simulink model "Autotrans_shift_test"  (R2022a)
settings: Solver=VariableStepAuto  StartTime=0.0  StopTime=50.0  FixedStep=0.001  MinStep=0.0001  RelTol=1e-3
model workspace (MATLAB code in the model file):
  | load sldemo_autotrans_data; %load initial conditions and other necessary data
undefined symbols (not defined in the file or in its folder): converter_data, downtab, emap, Hecate_param1, Hecate_param2, Hecate_param3, Hecate_param4, Iei, uptab, vehicledata
settings Model: DataTypeOverride=Double  MinMaxOverflowLogging=ForceOff  SimulationMode=accelerator  ExtModeTrigMode=oneshot  ExtModeArmWhenConnect=off  LastModifiedBy=fedformi_new
settings DataIOCC: TimeSaveName=Time_output_test345
settings OptimizationCC: BlockReduction=off  BooleanDataType=off
settings DebuggingCC: SaveWithParameterizedLinksMsg=none  UnderspecifiedInitializationDetection=Classic  MergeDetectMultiDrivingBlocksExec=none  SignalResolutionControl=TryResolveAllWithWarning
settings HardwareCC: TargetUnknown=on
settings ModelReferenceCC: PropagateSignalLabelsOutOfModel=off

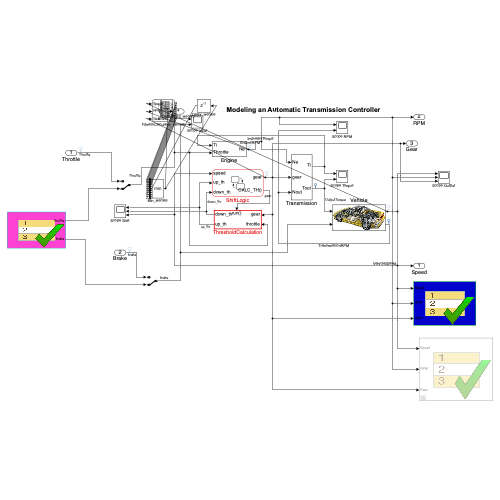
[thumbnail: Simulink's stored preview of the top-level diagram]
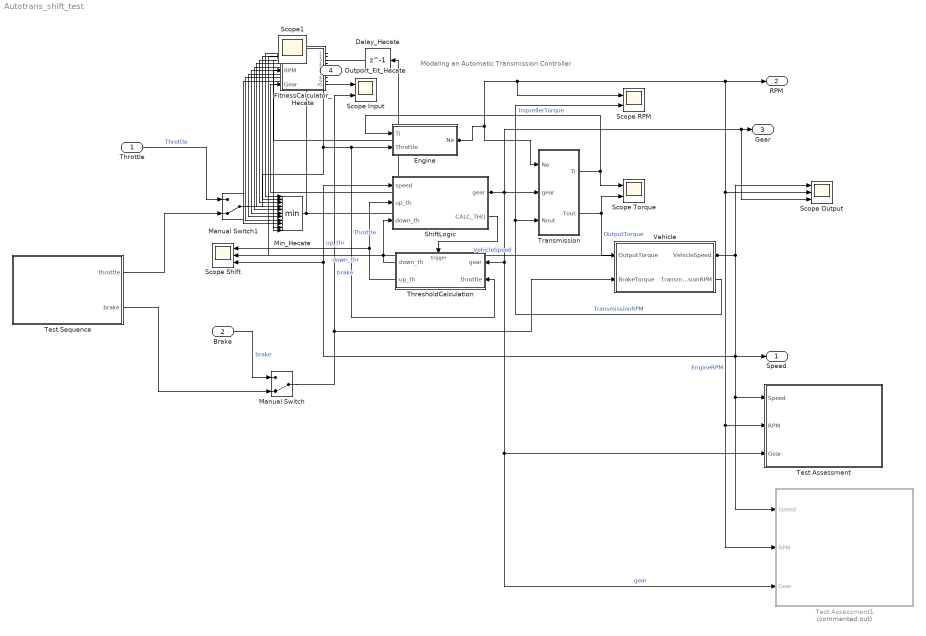
== system Autotrans_shift_test ==
  note: Modeling an Automatic Transmission Controller
  Throttle : Inport  Interpolate=off
  Brake : Inport  Port=2  Interpolate=off
  Delay_Hecate : Delay  DelayLength=1  InitialCondition=Inf
  Engine : Subsystem
  FitnessCalculator_Hecate : Stateflow chart  TreatAsAtomicUnit=on
  Manual Switch : ManualSwitch  CurrentSetting=0
  Manual Switch1 : ManualSwitch  CurrentSetting=0
  Min_Hecate : MinMax  Inputs=11
  Scope Input : Scope  NumInputPorts=2
  Scope Output : Scope  NumInputPorts=3
  Scope RPM : Scope  NumInputPorts=2
  Scope Shift : Scope  NumInputPorts=3
  Scope Torque : Scope  NumInputPorts=2
  ShiftLogic : Stateflow chart  TreatAsAtomicUnit=on
  Test Assessment : Test Sequence
  Test Assessment1 : Test Sequence  Commented=on  TreatAsAtomicUnit=on
  Test Sequence : Test Sequence  TreatAsAtomicUnit=on
  ThresholdCalculation : Subsystem  TreatAsAtomicUnit=on
  Transmission : Subsystem
  Vehicle : Subsystem  mask(vehicle model){Rfd=vehicledata(1), rload0=vehicledata(2), rload2=vehicledata(3), Rw=vehicledata(4), Iv=vehicledata(5), N20=vehicledata(6)/vehicledata(4)*vehicledata(1)}
      mask prompts: Rfd "final drive ratio"; rload0 "drag friction at wheels"; rload2 "aerodynamic drag"; Rw "wheel radius"; Iv "vehicle inertia"; N20 "initial transmission output speed"
      mask help: vehicle dynamics: torque input from trans., outputs are input speed (transmission output) and vehicle speed
      mask Display: image(imread([matlabroot,'/toolbox/simulink/simdemos/automotive/html/NSX_3Colors.jpg']))
  Speed : Outport  VectorParamsAs1DForOutWhenUnconnected=off
  RPM : Outport  Port=2  VectorParamsAs1DForOutWhenUnconnected=off
  Gear : Outport  Port=3  VectorParamsAs1DForOutWhenUnconnected=off
  Outport_Fit_Hecate : Outport  Port=4
  Scope1 : Scope
  wires:
  Transmission/1(Ti) -> Engine/1(Ti), Scope Torque/1  "ImprellerTorque"
  Engine/1(Ne) -> Transmission/1(Ne), Test Assessment1/2(RPM), Test Assessment/2(RPM), Scope Output/2, RPM/1, Scope RPM/1, FitnessCalculator_Hecate/2(RPM)  "EngineRPM"
  Vehicle/2(TransmissionRPM) -> Transmission/3(Nout), Scope RPM/2  "TransmissionRPM"
  ThresholdCalculation/1(down_th) -> Scope Shift/2, ShiftLogic/3(down_th)  "down_thr"
  ThresholdCalculation/2(up_th) -> ShiftLogic/2(up_th), Scope Shift/1  "up_thr"
  ShiftLogic/1(gear) -> ThresholdCalculation/1(gear), Test Assessment/3(Gear), Test Assessment1/3(Gear), Gear/1, Scope Output/3, Transmission/2(gear), FitnessCalculator_Hecate/3(Gear)  "gear"
  ShiftLogic/2(CALC_TH()) -> ThresholdCalculation/Trigger
  Vehicle/1(VehicleSpeed) -> Test Assessment1/1(Speed), Test Assessment/1(Speed), Speed/1, Scope Shift/3, ShiftLogic/1(speed), Scope Output/1, FitnessCalculator_Hecate/1(Speed)  "VehicleSpeed"
  Manual Switch1/1 -> ThresholdCalculation/2(throttle), Engine/2(Throttle), Scope Input/1  "Throttle"
  Transmission/2(Tout) -> Vehicle/1(OutputTorque), Scope Torque/2  "OutputTorque"
  Manual Switch/1 -> Vehicle/2(BrakeTorque), Scope Input/2  "brake"
  Test Sequence/1(throttle) -> Manual Switch1/2
  Test Sequence/2(brake) -> Manual Switch/2
  Brake/1 -> Manual Switch/1  "brake"
  Throttle/1 -> Manual Switch1/1  "Throttle"
  FitnessCalculator_Hecate/1(fitness_1) -> Min_Hecate/1
  FitnessCalculator_Hecate/2(fitness_2) -> Min_Hecate/2
  FitnessCalculator_Hecate/3(fitness_3) -> Min_Hecate/3
  FitnessCalculator_Hecate/4(fitness_4) -> Min_Hecate/4
  FitnessCalculator_Hecate/5(fitness_5) -> Min_Hecate/5
  FitnessCalculator_Hecate/6(fitness_6) -> Min_Hecate/6
  FitnessCalculator_Hecate/7(fitness_7) -> Min_Hecate/7
  FitnessCalculator_Hecate/8(fitness_8) -> Min_Hecate/8
  FitnessCalculator_Hecate/9(fitness_9) -> Min_Hecate/9
  FitnessCalculator_Hecate/10(fitness_10) -> Min_Hecate/10
  Min_Hecate/1 -> Delay_Hecate/1, Outport_Fit_Hecate/1
  Delay_Hecate/1 -> Min_Hecate/11

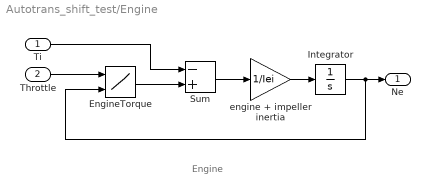
== system Autotrans_shift_test/Engine ==
  note: Engine
  Ti : Inport
  Throttle : Inport  Port=2
  EngineTorque : Lookup2D  RowIndex=thvec  ColumnIndex=nevec  Table=emap  SaturateOnIntegerOverflow=off
  Integrator : Integrator  InitialCondition=1000  LimitOutput=on  UpperSaturationLimit=6000  LowerSaturationLimit=600  ZeroCross=off
  Sum : Sum  Inputs=-+  InputSameDT=on  SaturateOnIntegerOverflow=on  OutDataTypeStr=Inherit: Same as first input
  engine + impeller inertia : Gain  Gain=1/Iei  SaturateOnIntegerOverflow=on  OutDataTypeStr=Inherit: Same as input  ParamDataTypeStr=Inherit: Same as input
  Ne : Outport  InitialOutput=0  VectorParamsAs1DForOutWhenUnconnected=off
  wires:
  Ti/1 -> Sum/1
  Throttle/1 -> EngineTorque/1
  Integrator/1 -> EngineTorque/2, Ne/1
  Sum/1 -> engine + impeller inertia/1
  engine + impeller inertia/1 -> Integrator/1
  EngineTorque/1 -> Sum/2

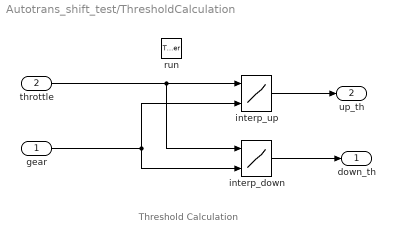
== system Autotrans_shift_test/ThresholdCalculation ==
  note: Threshold Calculation
  gear : Inport
  throttle : Inport  Port=2
  run : TriggerPort  TriggerType=function-call  VariantControl=(inherit)  ZeroCross=off
  interp_down : Lookup2D  RowIndex=downth  ColumnIndex=[1:4]  Table=downtab  OutDataTypeStr=double  SaturateOnIntegerOverflow=off  InputSameDT=off
      settings: LockScale=on
  interp_up : Lookup2D  RowIndex=upth  ColumnIndex=[1:4]  Table=uptab  OutDataTypeStr=double  SaturateOnIntegerOverflow=off  InputSameDT=off
      settings: LockScale=on
  down_th : Outport  VectorParamsAs1DForOutWhenUnconnected=off
  up_th : Outport  Port=2  VectorParamsAs1DForOutWhenUnconnected=off
  wires:
  interp_up/1 -> up_th/1
  interp_down/1 -> down_th/1
  throttle/1 -> interp_up/1, interp_down/1
  gear/1 -> interp_up/2, interp_down/2

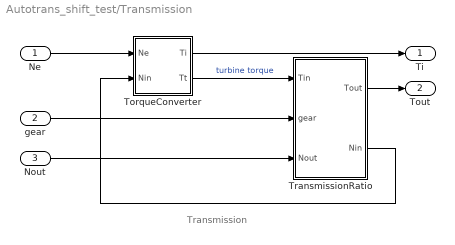
== system Autotrans_shift_test/Transmission ==
  note: Transmission
  Ne : Inport
  gear : Inport  Port=2
  Nout : Inport  Port=3
  TorqueConverter : Subsystem  mask(torque converter){speedratio=converter_data(:,1), Kfactor=converter_data(:,2), Torkratio=converter_data(:,3)}
      mask prompts: speedratio "speed ratio"; Kfactor "K factor"; Torkratio "torque ratio"
      mask help: torque converter
      mask Help: Torque converter input and output torques are computed as a function of the input and output speeds
      mask Display: plot([cos([90:10:450]*pi/180),.63*cos([90:10:450]*pi/180),.63*cos([90:10:240]*pi/180),cos([240:10:300]*pi/180),.63*cos([300]*pi/180)],[sin([90:10:450]*pi/180),.63*sin([90:10:450]*pi/180)+.1,.63*sin([90:10:240]*pi/180)+.1,sin([240:10:300]*pi/180),.63*sin([300]*pi/180)+.1])
  TransmissionRatio : Subsystem
  Ti : Outport  InitialOutput=0  VectorParamsAs1DForOutWhenUnconnected=off
  Tout : Outport  Port=2  InitialOutput=0  VectorParamsAs1DForOutWhenUnconnected=off
  wires:
  TransmissionRatio/1(Tout) -> Tout/1
  TorqueConverter/1(Ti) -> Ti/1
  Nout/1 -> TransmissionRatio/3(Nout)
  gear/1 -> TransmissionRatio/2(gear)
  Ne/1 -> TorqueConverter/1(Ne)
  TransmissionRatio/2(Nin) -> TorqueConverter/2(Nin)
  TorqueConverter/2(Tt) -> TransmissionRatio/1(Tin)  "turbine torque"

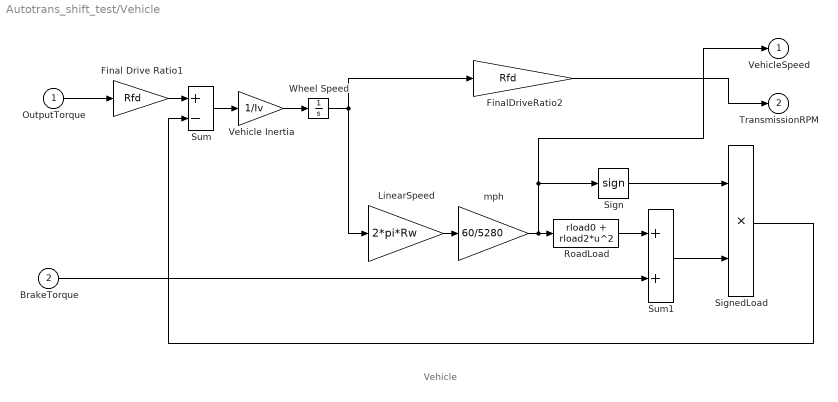
== system Autotrans_shift_test/Vehicle ==
  note: Vehicle
  OutputTorque : Inport
  BrakeTorque : Inport  Port=2
  Final Drive Ratio1 : Gain  Gain=Rfd  SaturateOnIntegerOverflow=on  OutDataTypeStr=Inherit: Same as input  ParamDataTypeStr=Inherit: Same as input
  FinalDriveRatio2 : Gain  Gain=Rfd  SaturateOnIntegerOverflow=on  OutDataTypeStr=Inherit: Same as input  ParamDataTypeStr=Inherit: Same as input
  LinearSpeed : Gain  Gain=2*pi*Rw  SaturateOnIntegerOverflow=on  OutDataTypeStr=Inherit: Same as input  ParamDataTypeStr=Inherit: Same as input
  RoadLoad : Fcn  Expr=rload0 + rload2*u^2
  Sign : Signum
  SignedLoad : Product  InputSameDT=on  SaturateOnIntegerOverflow=on  OutDataTypeStr=Inherit: Same as first input
  Sum : Sum  Inputs=+-  InputSameDT=on  SaturateOnIntegerOverflow=on  OutDataTypeStr=Inherit: Same as first input
  Sum1 : Sum  InputSameDT=on  SaturateOnIntegerOverflow=on  OutDataTypeStr=Inherit: Same as first input
  Vehicle Inertia : Gain  Gain=1/Iv  SaturateOnIntegerOverflow=on  OutDataTypeStr=Inherit: Same as input  ParamDataTypeStr=Inherit: Same as input
  Wheel Speed : Integrator  InitialCondition=N20/Rfd  ZeroCross=off
  mph : Gain  Gain=60/5280  SaturateOnIntegerOverflow=on  OutDataTypeStr=Inherit: Same as input  ParamDataTypeStr=Inherit: Same as input
  VehicleSpeed : Outport  InitialOutput=0  VectorParamsAs1DForOutWhenUnconnected=off
  TransmissionRPM : Outport  Port=2  InitialOutput=0  VectorParamsAs1DForOutWhenUnconnected=off
  wires:
  FinalDriveRatio2/1 -> TransmissionRPM/1
  BrakeTorque/1 -> Sum1/2
  Sum1/1 -> SignedLoad/2
  RoadLoad/1 -> Sum1/1
  Sign/1 -> SignedLoad/1
  SignedLoad/1 -> Sum/2
  OutputTorque/1 -> Final Drive Ratio1/1
  Vehicle Inertia/1 -> Wheel Speed/1
  Sum/1 -> Vehicle Inertia/1
  mph/1 -> VehicleSpeed/1, Sign/1, RoadLoad/1
  LinearSpeed/1 -> mph/1
  Wheel Speed/1 -> LinearSpeed/1, FinalDriveRatio2/1
  Final Drive Ratio1/1 -> Sum/1

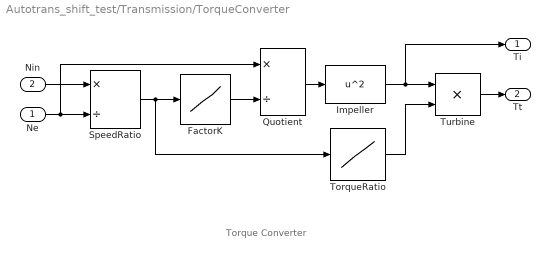
== system Autotrans_shift_test/Transmission/TorqueConverter ==
  note: Torque Converter
  Ne : Inport
  Nin : Inport  Port=2
  FactorK : Lookup  InputValues=speedratio  Table=Kfactor
  Impeller : Fcn  Expr=u^2
  Quotient : Product  Inputs=*/  InputSameDT=on  SaturateOnIntegerOverflow=on  OutDataTypeStr=Inherit: Same as first input
  SpeedRatio : Product  Inputs=*/  InputSameDT=on  SaturateOnIntegerOverflow=on  OutDataTypeStr=Inherit: Same as first input
  TorqueRatio : Lookup  InputValues=speedratio  Table=Torkratio
  Turbine : Product  InputSameDT=on  SaturateOnIntegerOverflow=on  OutDataTypeStr=Inherit: Same as first input
  Ti : Outport  InitialOutput=0  VectorParamsAs1DForOutWhenUnconnected=off
  Tt : Outport  Port=2  InitialOutput=0  VectorParamsAs1DForOutWhenUnconnected=off
  wires:
  TorqueRatio/1 -> Turbine/2
  Quotient/1 -> Impeller/1
  FactorK/1 -> Quotient/2
  SpeedRatio/1 -> TorqueRatio/1, FactorK/1
  Impeller/1 -> Turbine/1, Ti/1
  Turbine/1 -> Tt/1
  Ne/1 -> SpeedRatio/2, Quotient/1
  Nin/1 -> SpeedRatio/1

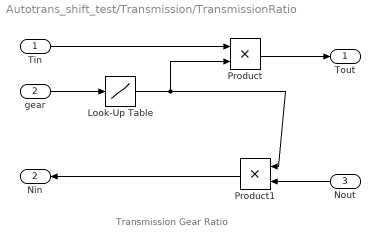
== system Autotrans_shift_test/Transmission/TransmissionRatio ==
  note: Transmission Gear Ratio
  Tin : Inport
  gear : Inport  Port=2
  Nout : Inport  Port=3
  Look-Up Table : Lookup  InputValues=[1 2 3 4]  Table=[2.393 1.450 1.000 0.677]  OutDataTypeStr=double  LockScale=on
  Product : Product  InputSameDT=on  SaturateOnIntegerOverflow=on  OutDataTypeStr=Inherit: Same as first input
  Product1 : Product  InputSameDT=on  SaturateOnIntegerOverflow=on  OutDataTypeStr=Inherit: Same as first input
  Tout : Outport  InitialOutput=0  VectorParamsAs1DForOutWhenUnconnected=off
  Nin : Outport  Port=2  InitialOutput=0  VectorParamsAs1DForOutWhenUnconnected=off
  wires:
  Look-Up Table/1 -> Product1/1, Product/2
  Nout/1 -> Product1/2
  Product1/1 -> Nin/1
  Product/1 -> Tout/1
  Tin/1 -> Product/1
  gear/1 -> Look-Up Table/1

== stateflow chart Autotrans_shift_test/Test Assessment1 ==
  state step_1
    verify(Speed >= 20)
    state step_1_1
      verify(Speed <= 30)
    state step_1_2
      verify(Speed <= 60)
    state step_1_3
      verify(1<=1)
      state step_1_3_1
        verify(Speed <= 80)
      state step_1_3_2
        verify(Speed <= 90)
        verify(Speed*30 >= RPM)
      state step_1_3_3
        verify(Speed <= 100)
        state step_1_3_2_1
          verify(Speed/20 > RPM/1000-Gear)
        state step_1_3_2_2
          verify(Speed/20 < RPM/1000+Gear)
        (default) -> (junction 99)
        step_1_3_3 -> (junction 99)
        (junction 99) -> (junction 100) [order 1] : [Speed <= 60
            | ]
        (junction 100) -> step_1_3_2_1 [order 1] : [~in(step_1.step_1_3.step_1_3_3.step_1_3_2_1)]
        (junction 100) -> (junction 103) [order 2]
        (junction 109) -> (junction 110)
        (junction 110) -> step_1_3_2_2 [order 1] : [~in(step_1.step_1_3.step_1_3_3.step_1_3_2_2)]
        (junction 110) -> (junction 113) [order 2]
        (junction 99) -> (junction 109) [order 2]
      (junction 91) -> (junction 94) [order 2]
      (junction 82) -> (junction 90) [order 2]
      (default) -> (junction 73)
      step_1_3 -> (junction 73)
      (junction 73) -> (junction 74) [order 1] : [RPM <= 3000
          | ]
      (junction 74) -> step_1_3_1 [order 1] : [~in(step_1.step_1_3.step_1_3_1)]
      (junction 73) -> (junction 82) [order 2]
      (junction 74) -> (junction 77) [order 2]
      (junction 82) -> (junction 83) [order 1] : [RPM <= 4000
          | ]
      (junction 83) -> step_1_3_2 [order 1] : [~in(step_1.step_1_3.step_1_3_2)]
      (junction 83) -> (junction 86) [order 2]
      (junction 90) -> (junction 91)
      (junction 91) -> step_1_3_3 [order 1] : [~in(step_1.step_1_3.step_1_3_3)]
    state step_1_4
      verify(Speed <= 150)
    step_1 -> (junction 47)
    (default) -> (junction 47)
    (junction 47) -> (junction 48) [order 1] : [Gear == 1
        | ]
    (junction 48) -> step_1_1 [order 1] : [~in(step_1.step_1_1)]
    (junction 47) -> (junction 56) [order 2]
    (junction 48) -> (junction 51) [order 2]
    (junction 56) -> (junction 57) [order 1] : [Gear == 2
        | ]
    (junction 57) -> step_1_2 [order 1] : [~in(step_1.step_1_2)]
    (junction 56) -> (junction 64) [order 2]
    (junction 57) -> (junction 60) [order 2]
    (junction 64) -> (junction 65) [order 1] : [Gear == 3
        | ]
    (junction 65) -> step_1_3 [order 1] : [~in(step_1.step_1_3)]
    (junction 65) -> (junction 68) [order 2]
    (junction 117) -> (junction 118)
    (junction 118) -> step_1_4 [order 1] : [~in(step_1.step_1_4)]
    (junction 118) -> (junction 121) [order 2]
    (junction 64) -> (junction 117) [order 2]
  (default) -> step_1
  data: Speed input; RPM input; Gear input

== stateflow chart Autotrans_shift_test/Test Sequence ==
  state Accelerate
    throttle = 100-Hecate_param1;
    % Random comment;
    brake = 0+Hecate_param2;
  state Constant_speed
    throttle = 0;
    brake = 0+Hecate_param4;
  (default) -> Accelerate
  Accelerate -> Constant_speed : [
      | after(20-Hecate_param3,sec)
      | ]
  data: throttle output; brake output; Hecate_param1 parameter; Hecate_param2 parameter; Hecate_param3 parameter; Hecate_param4 parameter

== stateflow chart Autotrans_shift_test/FitnessCalculator_Hecate ==
  state step_1
    fitness_1 = Inf;
    fitness_2 = Inf;
    fitness_3 = Inf;
    fitness_4 = Inf;
    fitness_5 = Inf;
    fitness_6 = Inf;
    fitness_7 = Inf;
    fitness_8 = Inf;
    fitness_9 = Inf;
    fitness_10 = Inf;
    state step_1_1
      fitness_1 = min([3000-(RPM);2-(Gear);Speed-(70);]);
      fitness_2 = max([70-(Speed);Gear-(3);Speed-(45);]);
      fitness_3 = Inf;
      fitness_4 = Inf;
      fitness_5 = Inf;
      fitness_6 = Inf;
      fitness_7 = Inf;
      fitness_8 = Inf;
      fitness_9 = Inf;
      fitness_10 = Inf;
      state step_1_1_1
        fitness_1 = min([3000-(RPM);2-(Gear);Speed-(70);]);
        fitness_2 = max([70-(Speed);Gear-(3);Speed-(45);]);
        fitness_3 = 50-(Speed);
        fitness_4 = Inf;
        fitness_5 = Inf;
        fitness_6 = Inf;
        fitness_7 = Inf;
        fitness_8 = Inf;
        fitness_9 = Inf;
        fitness_10 = Inf;
      state step_1_1_2
        fitness_1 = min([3000-(RPM);2-(Gear);Speed-(70);]);
        fitness_2 = max([70-(Speed);Gear-(3);Speed-(45);]);
        fitness_3 = Inf;
        fitness_4 = Speed-(60);
        fitness_5 = Inf;
        fitness_6 = Inf;
        fitness_7 = Inf;
        fitness_8 = Inf;
        fitness_9 = Inf;
        fitness_10 = Inf;
      (default) -> step_1_1_1
      step_1_1_2 -> step_1_1_1 : [RPM < 2900]
      step_1_1_1 -> step_1_1_2 : [RPM >= 3300]
    state step_1_2
      fitness_1 = Inf;
      fitness_2 = Inf;
      fitness_3 = Inf;
      fitness_4 = Inf;
      fitness_5 = 3500-(RPM);
      fitness_6 = Inf;
      fitness_7 = Inf;
      fitness_8 = Inf;
      fitness_9 = Inf;
      fitness_10 = Inf;
    state step_1_3
      fitness_1 = Inf;
      fitness_2 = Inf;
      fitness_3 = Inf;
      fitness_4 = Inf;
      fitness_5 = Inf;
      fitness_6 = 4000-(RPM);
      fitness_7 = Inf;
      fitness_8 = Inf;
      fitness_9 = Inf;
      fitness_10 = Inf;
    (default) -> (junction 4)
    step_1_3 -> (junction 4) : [(Gear <= 2)|(Gear == 3)]
    step_1_2 -> (junction 4) : [(Gear <= 2)|~(Gear == 3)]
    (junction 4) -> step_1_1 [order 1] : [Gear <= 2]
    (junction 4) -> step_1_2 [order 2] : [Gear == 3]
    (junction 4) -> step_1_3 [order 3] : []
    step_1_1 -> (junction 4) : [~(Gear <= 2)]
  state step_2
    fitness_1 = Inf;
    fitness_2 = Inf;
    fitness_3 = Inf;
    fitness_4 = Inf;
    fitness_5 = Inf;
    fitness_6 = Inf;
    fitness_7 = Inf;
    fitness_8 = Inf;
    fitness_9 = Inf;
    fitness_10 = Inf;
    state step_2_2
      fitness_1 = Inf;
      fitness_2 = Inf;
      fitness_3 = Inf;
      fitness_4 = Inf;
      fitness_5 = Inf;
      fitness_6 = Inf;
      fitness_7 = Inf;
      fitness_8 = Inf;
      fitness_9 = Inf;
      fitness_10 = Inf;
      state step_2_2_1
        fitness_1 = Inf;
        fitness_2 = Inf;
        fitness_3 = Inf;
        fitness_4 = Inf;
        fitness_5 = Inf;
        fitness_6 = Inf;
        fitness_7 = Inf;
        fitness_8 = 100-(Speed);
        fitness_9 = Inf;
        fitness_10 = Inf;
      state step_2_2_2
        fitness_1 = Inf;
        fitness_2 = Inf;
        fitness_3 = Inf;
        fitness_4 = Inf;
        fitness_5 = Inf;
        fitness_6 = Inf;
        fitness_7 = Inf;
        fitness_8 = Inf;
        fitness_9 = Speed-(110);
        fitness_10 = Inf;
      (default) -> (junction 22)
      step_2_2_2 -> (junction 22) : [(RPM < 3700)]
      step_2_2_1 -> (junction 22) : [~(RPM < 3700)]
      (junction 22) -> step_2_2_1 [order 1] : [RPM < 3700]
      (junction 22) -> step_2_2_2 [order 2] : []
    state step_2_1
      fitness_1 = Inf;
      fitness_2 = Inf;
      fitness_3 = Inf;
      fitness_4 = Inf;
      fitness_5 = Inf;
      fitness_6 = Inf;
      fitness_7 = 90-(Speed);
      fitness_8 = Inf;
      fitness_9 = Inf;
      fitness_10 = Inf;
    (default) -> step_2_1
    step_2_2 -> step_2_1 : [true]
    step_2_1 -> step_2_2 : [after(2, sec) && Gear == 4]
  state step_3
    fitness_1 = Inf;
    fitness_2 = Inf;
    fitness_3 = Inf;
    fitness_4 = Inf;
    fitness_5 = Inf;
    fitness_6 = Inf;
    fitness_7 = Inf;
    fitness_8 = Inf;
    fitness_9 = Inf;
    fitness_10 = Speed-(70);
  (default) -> step_1
  step_1 -> step_3 [order 1] : [Speed > 120]
  step_1 -> step_2 [order 2] : [after(25, sec)]
  step_2 -> step_3 : [after(20, sec)]
  data: Speed input; RPM input; Gear input; fitness_1 output; fitness_2 output; fitness_3 output; fitness_4 output; fitness_5 output; fitness_6 output; fitness_7 output; fitness_8 output; fitness_9 output; fitness_10 output

== stateflow chart Autotrans_shift_test/ShiftLogic ==
  settings: updateMethod=DISCRETE  sampleTime=0.04
  state gear_state [parallel]
    settings: executionOrder=1
    state fourth
      entry:
      gear = 4;
    state third
      entry:
      gear = 3;
    state second
      entry:
      gear = 2;
    state first
      entry:
      gear = 1;
    (default) -> first
    second -> third [order 1] : UP
    first -> second : UP
    third -> fourth [order 1] : UP
    second -> first [order 2] : DOWN
    fourth -> third : DOWN
    third -> second [order 2] : DOWN
  state selection_state [parallel]
    during: CALC_TH;
    settings: executionOrder=2
    state steady_state
    state upshifting
    state downshifting
    (default) -> steady_state
    steady_state -> upshifting [order 1] : [speed > up_th]
    steady_state -> downshifting [order 2] : [speed < down_th]
    downshifting -> steady_state [order 1] : after(TWAIT,tick)
        | [speed <= down_th]
        | {gear_state.DOWN}
    downshifting -> steady_state [order 2] : [speed > down_th]
    upshifting -> steady_state [order 1] : after(TWAIT,tick)
        | [speed >= up_th]
        | {gear_state.UP}
    upshifting -> steady_state [order 2] : [speed < up_th]
  data: speed input double; gear output fixdt(0,8,5) [1..4]; TWAIT parameter fixdt(0,8,6); up_th input double; down_th input double
  events: DOWN local EITHER_EDGE_EVENT; UP local EITHER_EDGE_EVENT; CALC_TH output FUNCTION_CALL_EVENT

== stateflow chart Autotrans_shift_test/Test Assessment ==
  state Scenario_1
    state Group1
      verify(Speed >= 0)
      state AT2
        verify(Speed < 120)
        state AT2_1
          verify(RPM<6000)
          verify(Speed >= 35)
        (default) -> AT2_1
      state ATend
        verify(Gear < 5)
      (junction 118) -> (junction 121) [order 2]
      (junction 108) -> (junction 117) [order 2]
      (default) -> (junction 108)
      Group1 -> (junction 108) [order 1]
      (junction 108) -> (junction 109) [order 1] : [RPM > 2500
          | ]
      (junction 109) -> AT2 [order 1] : [~in(Scenario_1.Group1.AT2)]
      (junction 109) -> (junction 112) [order 2]
      (junction 117) -> (junction 118)
      (junction 118) -> ATend [order 1] : [~in(Scenario_1.Group1.ATend)]
    state Group2
      verify(RPM >= 600)
    state Group3
      verify(Gear >= 0)
    (default) -> Group1
    Group1 -> (junction 564) [order 2] : [
        | t >= 10 && Gear >= 4
        | ]
    (junction 564) -> (junction 170)
    Group1 -> Group2 [order 1] : [
        | t >= 20
        | ]
    (junction 170) -> Group3
  state Scenario_2
    state step_1
      state step_1_1
        state step_1_1_1
          verify(RPM > 3000)
        state step_1_1_2
        (default) -> (junction 587)
        Scenario_2.step_1.step_1_1 -> (junction 587)
        (junction 587) -> (junction 588) [order 1] : [Speed-(RPM/1000)^Gear > 35 || t < 20
            | ]
        (junction 588) -> Scenario_2.step_1.step_1_1.step_1_1_1 [order 1] : [~in(Scenario_2.step_1.step_1_1.step_1_1_1)]
        (junction 588) -> (junction 591) [order 2]
        (junction 596) -> (junction 597)
        (junction 597) -> Scenario_2.step_1.step_1_1.step_1_1_2 [order 1] : [~in(Scenario_2.step_1.step_1_1.step_1_1_2)]
        (junction 597) -> (junction 600) [order 2]
        (junction 587) -> (junction 596) [order 2]
      state step_1_2
      (default) -> (junction 573)
      Scenario_2.step_1 -> (junction 573)
      (junction 573) -> (junction 574) [order 1] : [Speed <= 70 && hasChangedTo(Gear,2)
          | ]
      (junction 574) -> Scenario_2.step_1.step_1_1 [order 1] : [~in(Scenario_2.step_1.step_1_1)]
      (junction 574) -> (junction 577) [order 2]
      (junction 604) -> (junction 605)
      (junction 605) -> Scenario_2.step_1.step_1_2 [order 1] : [~in(Scenario_2.step_1.step_1_2)]
      (junction 605) -> (junction 608) [order 2]
      (junction 573) -> (junction 604) [order 2]
    (default) -> Scenario_2.step_1
  state Scenario_3
    state step_1
      state step_1_1
        verify(RPM < 3000 && Gear <= 2 & Speed > 70) % Random comment
        verify(Speed < 70 || Gear > 3 || Speed > 45)
        state step_1_1_1
          verify(Speed < 50)
        state step_1_1_2
          verify(Speed >= 60)
        (default) -> Scenario_3.step_1.step_1_1.step_1_1_1
        Scenario_3.step_1.step_1_1.step_1_1_1 -> Scenario_3.step_1.step_1_1.step_1_1_2 : [
            | RPM >= 3300
            | ]
        Scenario_3.step_1.step_1_1.step_1_1_2 -> Scenario_3.step_1.step_1_1.step_1_1_1 : [
            | RPM < 2900
            | ]
      state step_1_2
        verify(RPM <= 3500)
      state step_1_3
        verify(RPM < 4000)
      (default) -> (junction 206)
      Scenario_3.step_1 -> (junction 206) [order 1]
      (junction 206) -> (junction 207) [order 1] : [Gear <= 2
          | ]
      (junction 207) -> Scenario_3.step_1.step_1_1 [order 1] : [~in(Scenario_3.step_1.step_1_1)]
      (junction 206) -> (junction 223) [order 2]
      (junction 207) -> (junction 210) [order 2]
      (junction 223) -> (junction 224) [order 1] : [Gear == 3
          | ]
      (junction 224) -> Scenario_3.step_1.step_1_2 [order 1] : [~in(Scenario_3.step_1.step_1_2)]
      (junction 223) -> (junction 231) [order 2]
      (junction 224) -> (junction 227) [order 2]
      (junction 231) -> (junction 232)
      (junction 232) -> Scenario_3.step_1.step_1_3 [order 1] : [~in(Scenario_3.step_1.step_1_3)]
      (junction 232) -> (junction 235) [order 2]
    state step_2
      state step_2_1
        verify(Speed < 90)
      state step_2_2
        state step_2_2_1
          verify(Speed < 100)
        state step_2_2_2
          verify(Speed >= 110)
        (default) -> (junction 248)
        Scenario_3.step_2.step_2_2 -> (junction 248) [order 1]
        (junction 248) -> (junction 249) [order 1] : [RPM < 3700
            | ]
        (junction 249) -> Scenario_3.step_2.step_2_2.step_2_2_1 [order 1] : [~in(Scenario_3.step_2.step_2_2.step_2_2_1)]
        (junction 249) -> (junction 252) [order 2]
        (junction 257) -> (junction 258)
        (junction 258) -> Scenario_3.step_2.step_2_2.step_2_2_2 [order 1] : [~in(Scenario_3.step_2.step_2_2.step_2_2_2)]
        (junction 258) -> (junction 261) [order 2]
        (junction 248) -> (junction 257) [order 2]
      (default) -> Scenario_3.step_2.step_2_1
      Scenario_3.step_2.step_2_1 -> Scenario_3.step_2.step_2_2 : [
          | after(2, sec) && Gear == 4
          | ]
      Scenario_3.step_2.step_2_2 -> Scenario_3.step_2.step_2_1 [order 1]
    state step_3
      verify(Speed > 70)
    (default) -> Scenario_3.step_1
    Scenario_3.step_1 -> (junction 561) [order 1] : [
        | Speed > 120
        | ]
    (junction 561) -> (junction 199)
    Scenario_3.step_1 -> Scenario_3.step_2 [order 2] : [
        | after(25, sec)
        | ]
    Scenario_3.step_2 -> Scenario_3.step_3 : [
        | after(20, sec)
        | ]
    (junction 199) -> Scenario_3.step_3
  state Scenario_4
    state step_1
      verify(Speed >= 20)
      state step_1_1
        verify(Speed <= 30)
      state step_1_2
        verify(Speed <= 60)
      state step_1_3
        verify(true)
        state step_1_3_1
          verify(Speed <= 80)
        state step_1_3_3
          verify(Speed <= 90)
          verify(Speed*30 >= RPM)
        state step_1_3_2
          verify(Speed <= 100)
          state step_1_3_2_1
            verify(Speed > RPM/1000*Gear)
          state step_1_3_2_2
            verify(Speed < RPM/1000*Gear)
          (junction 380) -> (junction 383) [order 2]
          (junction 379) -> (junction 380) [order 1] : [(Speed <= 60)
              | ]
          (junction 380) -> step_1_3_2_1 [order 1] : [~in(Scenario_4.step_1.step_1_3.step_1_3_2.step_1_3_2_1)]
          (junction 368) -> (junction 369)
          (junction 369) -> step_1_3_2_2 [order 1] : [~in(Scenario_4.step_1.step_1_3.step_1_3_2.step_1_3_2_2)]
          (junction 369) -> (junction 372) [order 2]
          (junction 379) -> (junction 368) [order 2]
          step_1_3_2 -> (junction 379)
          (default) -> (junction 379)
        (junction 339) -> (junction 342) [order 2]
        (junction 303) -> (junction 338) [order 2]
        (default) -> (junction 303)
        Scenario_4.step_1.step_1_3 -> (junction 303)
        (junction 303) -> (junction 304) [order 1] : [(RPM <= 3000)
            | ]
        (junction 304) -> step_1_3_1 [order 1] : [~in(Scenario_4.step_1.step_1_3.step_1_3_1)]
        (junction 338) -> (junction 312) [order 2]
        (junction 304) -> (junction 307) [order 2]
        (junction 338) -> (junction 339) [order 1] : [(RPM <= 4000)
            | ]
        (junction 339) -> step_1_3_3 [order 1] : [~in(Scenario_4.step_1.step_1_3.step_1_3_3)]
        (junction 312) -> (junction 313)
        (junction 313) -> step_1_3_2 [order 1] : [~in(Scenario_4.step_1.step_1_3.step_1_3_2)]
        (junction 313) -> (junction 316) [order 2]
      state step_1_4
        verify(Speed <= 150)
      Scenario_4.step_1 -> (junction 281)
      (default) -> (junction 281)
      (junction 281) -> (junction 282) [order 1] : [(Gear == 1)
          | ]
      (junction 282) -> Scenario_4.step_1.step_1_1 [order 1] : [~in(Scenario_4.step_1.step_1_1)]
      (junction 281) -> (junction 321) [order 2]
      (junction 282) -> (junction 285) [order 2]
      (junction 321) -> (junction 322) [order 1] : [(Gear == 2)
          | ]
      (junction 322) -> Scenario_4.step_1.step_1_2 [order 1] : [~in(Scenario_4.step_1.step_1_2)]
      (junction 321) -> (junction 290) [order 2]
      (junction 322) -> (junction 325) [order 2]
      (junction 290) -> (junction 291) [order 1] : [(Gear == 3)
          | ]
      (junction 291) -> Scenario_4.step_1.step_1_3 [order 1] : [~in(Scenario_4.step_1.step_1_3)]
      (junction 290) -> (junction 329) [order 2]
      (junction 291) -> (junction 294) [order 2]
      (junction 329) -> (junction 330)
      (junction 330) -> step_1_4 [order 1] : [~in(Scenario_4.step_1.step_1_4)]
      (junction 330) -> (junction 333) [order 2]
    (default) -> Scenario_4.step_1
  state Scenario_5
    state step_1
      verify(false)
      state step_1_1
        verify(false)
        state step_1_1_1
          verify(false)
        state step_1_1_2
          verify(false)
        (default) -> Scenario_5.step_1.step_1_1.step_1_1_1
        Scenario_5.step_1.step_1_1.step_1_1_1 -> Scenario_5.step_1.step_1_1.step_1_1_2 : [
            | RPM >= 3300
            | ]
        Scenario_5.step_1.step_1_1.step_1_1_2 -> Scenario_5.step_1.step_1_1.step_1_1_1 : [
            | RPM < 2900
            | ]
      state step_1_2
        verify(false)
      state step_1_3
        verify(false)
      Scenario_5.step_1 -> (junction 485) [order 1]
      (default) -> (junction 485)
      (junction 485) -> (junction 486) [order 1] : [Gear <= 2
          | ]
      (junction 486) -> Scenario_5.step_1.step_1_1 [order 1] : [~in(Scenario_5.step_1.step_1_1)]
      (junction 485) -> (junction 500) [order 2]
      (junction 486) -> (junction 489) [order 2]
      (junction 500) -> (junction 501) [order 1] : [Gear == 3
          | ]
      (junction 501) -> Scenario_5.step_1.step_1_2 [order 1] : [~in(Scenario_5.step_1.step_1_2)]
      (junction 501) -> (junction 504) [order 2]
      (junction 508) -> (junction 509)
      (junction 509) -> Scenario_5.step_1.step_1_3 [order 1] : [~in(Scenario_5.step_1.step_1_3)]
      (junction 509) -> (junction 512) [order 2]
      (junction 500) -> (junction 508) [order 2]
    state step_2
      verify(false)
      state step_2_1
        verify(false)
      state step_2_2
        verify(false)
        state step_2_2_1
          verify(false)
        state step_2_2_2
          verify(false)
        (default) -> (junction 527)
        Scenario_5.step_2.step_2_2 -> (junction 527) [order 1]
        (junction 527) -> (junction 528) [order 1] : [RPM < 3700
            | ]
        (junction 528) -> Scenario_5.step_2.step_2_2.step_2_2_1 [order 1] : [~in(Scenario_5.step_2.step_2_2.step_2_2_1)]
        (junction 528) -> (junction 531) [order 2]
        (junction 536) -> (junction 537)
        (junction 537) -> Scenario_5.step_2.step_2_2.step_2_2_2 [order 1] : [~in(Scenario_5.step_2.step_2_2.step_2_2_2)]
        (junction 537) -> (junction 540) [order 2]
        (junction 527) -> (junction 536) [order 2]
      (default) -> Scenario_5.step_2.step_2_1
      Scenario_5.step_2.step_2_1 -> Scenario_5.step_2.step_2_2 : [
          | after(2, sec) && Gear == 4
          | ]
      Scenario_5.step_2.step_2_2 -> Scenario_5.step_2.step_2_1 [order 1] : [
          | RPM <= 3500
          | ]
    state step_3
      verify(false)
    (default) -> Scenario_5.step_1
    Scenario_5.step_1 -> (junction 558) [order 1] : [
        | Speed > 120
        | ]
    (junction 558) -> (junction 547)
    Scenario_5.step_1 -> Scenario_5.step_2 [order 2] : [
        | after(25, sec)
        | ]
    Scenario_5.step_2 -> Scenario_5.step_3 : [
        | after(20, sec)
        | ]
    (junction 547) -> Scenario_5.step_3
  state Scenario_6
    state step_1
      verify(hasChanged(Gear));
      verify(hasChanged(Speed));
      verify(hasChangedFrom(Gear,2));
      verify(hasChangedTo(Gear,2));
    (default) -> Scenario_6.step_1
  (default) -> Scenario_1 [order 1] : [Active_Scenario_Index == 1]
  (default) -> Scenario_2 [order 2] : [Active_Scenario_Index == 2]
  (default) -> Scenario_3 [order 3] : [Active_Scenario_Index == 3]
  (default) -> Scenario_4 [order 4] : [Active_Scenario_Index == 4]
  (default) -> Scenario_5 [order 5] : [Active_Scenario_Index == 5]
  (default) -> Scenario_6 [order 6] : {assert(Active_Scenario_Index == 6,'The value of Scenario Parameter ''Active_Scenario_Index'' is not valid. Use the index of the scenario to specify it.')}
  data: Speed input; RPM input; Gear input; Active_Scenario_Index parameter =3
